simulink model "zeroandhold_2017a"  (R2017a)
settings: Solver=FixedStepAuto  StartTime=0.0  StopTime=2  FixedStep=0.001  RelTol=1e-3
settings Model: Creator=Home  LastModifiedBy=Home

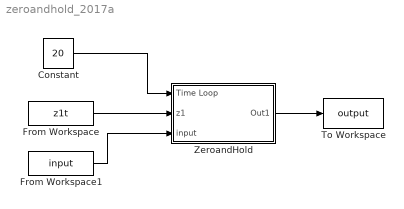
== system zeroandhold_2017a ==
  Constant : Constant  Value=20
  From Workspace : FromWorkspace  VariableName=z1t  SampleTime=0
  From Workspace1 : FromWorkspace  VariableName=input  SampleTime=0
  To Workspace : ToWorkspace  VariableName=output  SampleTime=-1
      settings: Save2DSignal=2-D array (concatenate along first dimension)
  ZeroandHold : Subsystem
  wires:
  Constant/1 -> ZeroandHold/1(Time Loop)
  From Workspace/1 -> ZeroandHold/2(z1)
  From Workspace1/1 -> ZeroandHold/3(input)
  ZeroandHold/1(Out1) -> To Workspace/1

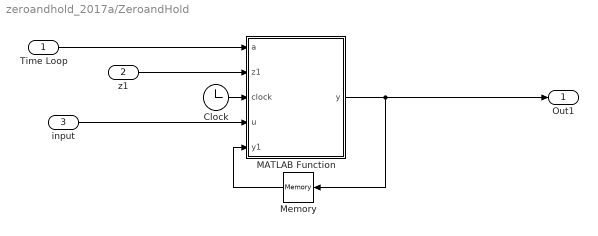
== system zeroandhold_2017a/ZeroandHold ==
  Time Loop : Inport
  z1 : Inport  Port=2
  input : Inport  Port=3
  Clock : Clock
  MATLAB Function : MATLAB Function  TreatAsAtomicUnit=on
  Memory : Memory
  Out1 : Outport
  wires:
  Clock/1 -> MATLAB Function/3(clock)
  z1/1 -> MATLAB Function/2(z1)
  input/1 -> MATLAB Function/4(u)
  MATLAB Function/1(y) -> Out1/1, Memory/1
  Memory/1 -> MATLAB Function/5(y1)
  Time Loop/1 -> MATLAB Function/1(a)

== matlab function zeroandhold_2017a/ZeroandHold/MATLAB Function ==
  data: a input; z1 input; clock input; u input; y output; y1 input
function y = fcn(a,z1,clock,u,y1)
dt = 0.001;
n = clock/dt;
if z1<0
    y =0;
else
if z1 == 0
n1 = n;
else
n1 = 100;
end
deln = n-n1;
if rem(deln,a)==0
y = u;
else
y = y1;
end
end
